simulink library "sm_excv_chassis_lib"  (R2026a)
settings: Solver=VariableStepAuto
undefined symbols (not defined in the file): Excv, Trac, track_seg_tgts_seg25i2u0r3, TracTrac, X, Y, Z
libraries: sm_lib x169, nesl_utility x12, $bdroot x8, sm_trackV_lib_chain_underc_elem x4
(part 1 of 4)
Description:
  | Copyright 2024-2026 The MathWorks, Inc.
settings Model: Creator=smiller  LastModifiedBy=smiller

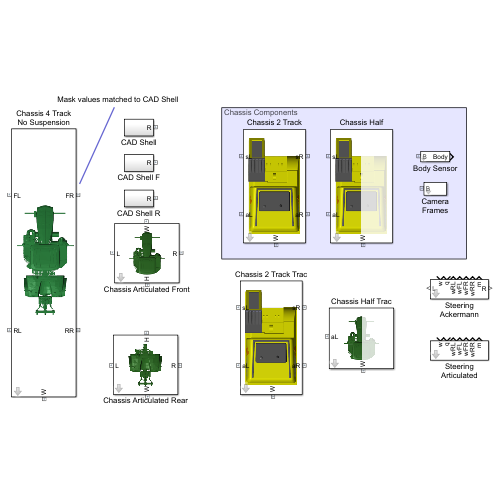
[thumbnail: Simulink's stored preview of the top-level diagram]
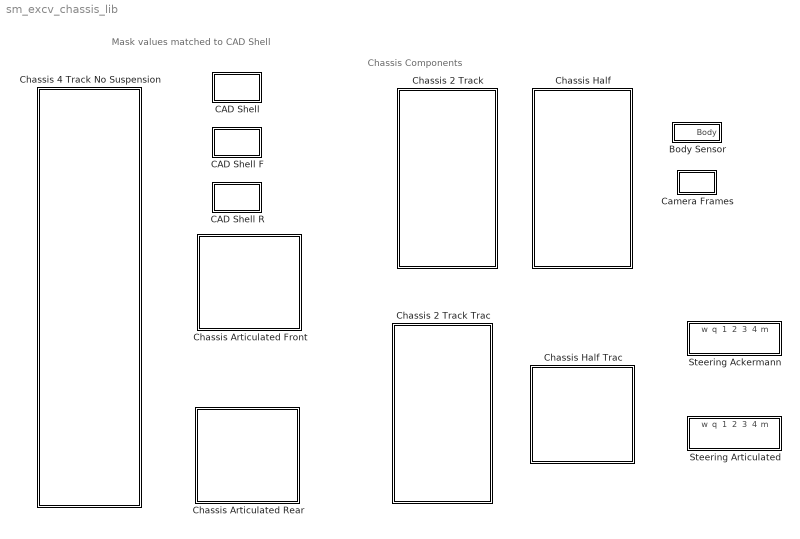
== system sm_excv_chassis_lib ==
  note: Mask values matched to CAD Shell
  note: Chassis Components
  Body Sensor : Subsystem  mask(Measurements in Body Frame){offset_body_sensor=[0 0 0]}
      mask prompts: offset_body_sensor "Sensor Frame Offset [x y z] (m)"
  CAD Shell : Subsystem
  CAD Shell F : Subsystem
  CAD Shell R : Subsystem
  Camera Frames : Subsystem  mask{Camera=Excv.Chassis.Camera}
      mask prompts: Camera "Camera Offsets (structure) (m)"
  Chassis 2 Track : Subsystem  mask{offset_cg=Excv.Chassis.CGOffset, offset_axle=Excv.Chassis.AxleOffset, offset_Lcyl=Excv.Chassis.SuspOffset, offset_sprk2axle_x=Excv.Frame.AxleX, offset_sprk2axle_y=Excv.Frame.AxleY, Camera=Excv.Chassis.Camera, track_sep_ctr=Excv.Chassis.TrackSepCtr, axle_rad=Excv.Chassis.AxleRad, axle_opc=0, chassis_mass=Excv.Chassis.Mass, chassis_moi=Excv.Chassis.MOI, chassis_poi=Excv.Chassis.POI, body_clr=[1 1 0], trim_clr=[0.4 0.4 0.4], accent_clr=[1 0.6 0], chassis_opc=1, cyl_len=Excv.Chassis.Susp.Cylinder.Cylinder.Len, cyl_rad=Excv.Chassis.Susp.Cylinder.Cylinder.Rad, cyl_mass=Excv.Chassis.Susp.Cylinder.Cylinder.Mass, piston_len=Excv.Chassis.Susp.Cylinder.Piston.Len, piston_rad=Excv.Chassis.Susp.Cylinder.Piston.Rad, piston_mass=Excv.Chassis.Susp.Cylinder.Piston.Mass, spr_k=Excv.Chassis.Susp.Cylinder.k, spr_d=Excv.Chassis.Susp.Cylinder.b, spr_xeq=Excv.Chassis.Susp.Cylinder.xeq}
      mask prompts: offset_cg "Offset to CG [long height lat] (m)"; offset_axle "Offset to Axle [long height lat] (m)"; offset_Lcyl "Offset to Left Cylinder [long height lat] (m)"; offset_sprk2axle_x "Offset Sprocket to Axle Long (m)"; offset_sprk2axle_y "Offset Sprocket to Axle Height (m)"; Camera "Camera Offsets (structure) (m)"; track_sep_ctr "Track Width (m)"; axle_rad "Axle Radius (m)"; axle_opc "Axle Opacity (0-1)"; chassis_mass "Chassis Mass (kg)"; chassis_moi "Chassis Moments of Inertia (kg*m^2)"; chassis_poi "Chassis Products of Inertia (kg*m^2)"; body_clr "Body Color [R G B] (0-1)"; trim_clr "Trim Color  [R G B] (0-1)"; accent_clr "Accent Color [R G B] (0-1)"; chassis_opc "Opacity (0-1)"; cyl_len "Cylinder Length (m)"; cyl_rad "Cylinder Radius (m)"; cyl_mass "Cylinder Mass (kg)"; piston_len "Piston Length (m)"; piston_rad "Piston Radius (m)"; piston_mass "Piston Mass (kg)"; spr_k "Stiffness (N/m)"; spr_d "Damping (N/(m/s))"; spr_xeq "Equilibrium Position (m)"
      settings: PortSchema="{\"entries\":[{\"content\":{\"sides\":[{\"content\":{\"connectorIds\":[\"LConn1\",\"LConn2\"]},\"type\":\"ConnectorPlacement.EquallySpacedRectSide\",\"uuid\":\"edd0f9cd-c75d-460e-8747-c453c06c3b51\"},{\"content\":{\"connectorIds\":[\"RConn1\",\"RConn2\"],\"side\":\"RIGHT\"},\"type\":\"ConnectorPlacement.EquallySpacedRectSide\",\"uuid\":\"aac0b74e-f978-42e3-a6a1-4bc72aaab1ab\"},{\"content\":{\"side\":\"TOP\"},\"type\":\"ConnectorPlacement.EquallySpacedRectSide\",\"uuid\":\"f25955ca-c2f5-46fd-b059-2b680dae975d\"},{\"content\":{\"connectorIds\":[\"RConn3\"],\"side\":\"BOTTOM\"},\"type\":\"ConnectorPlacement.EquallySpacedRectSide\",\"uuid\":\"7501e828-daf5-40c9-b971-42e639c94cdf\"}]},\"type\":\"ConnectorPlacement.EquallySpacedConnector\",\"uuid\":\"6826b738-8ce7-493d-aa91-65501067c2e5\"}],\"packageUris\":[\"http://schema.mathworks.com/mf0/Connector/R2020b\"],\"version\":\"1.0\"}"
      mask TypeOptions offset_cg:
      | Transform
      | Chassis Ref to CG/TranslationCartesianOffset
      mask TypeOptions offset_axle:
      | Transform
      | Chassis Ref
      | to Axle/TranslationCartesianOffset
      mask TypeOptions Camera:
      | Camera
      | Frames/Camera
      mask TypeOptions axle_rad: Axle/CylinderRadius
      mask TypeOptions axle_opc: Axle/GraphicOpacity
      mask TypeOptions chassis_mass:
      | Inertia
      | Chassis/Mass
      mask TypeOptions chassis_moi:
      | Inertia
      | Chassis/MomentsOfInertia
      mask TypeOptions chassis_poi:
      | Inertia
      | Chassis/ProductsOfInertia
      mask TypeOptions cyl_len:
      | Cylinder
      | Left/cyl_len | Cylinder
      | Right/cyl_len
      mask TypeOptions cyl_rad:
      | Cylinder
      | Left/cyl_rad | Cylinder
      | Right/cyl_rad
      mask TypeOptions cyl_mass:
      | Cylinder
      | Left/cyl_mass | Cylinder
      | Right/cyl_mass
      mask TypeOptions piston_len:
      | Cylinder
      | Left/piston_len | Cylinder
      | Right/piston_len
      mask TypeOptions piston_rad:
      | Cylinder
      | Left/piston_rad | Cylinder
      | Right/piston_rad
      mask TypeOptions piston_mass:
      | Cylinder
      | Left/piston_mass | Cylinder
      | Right/piston_mass
      mask TypeOptions spr_k:
      | Cylinder
      | Left/spr_k | Cylinder
      | Right/spr_k
      mask TypeOptions spr_d:
      | Cylinder
      | Left/spr_d | Cylinder
      | Right/spr_d
      mask TypeOptions spr_xeq:
      | Cylinder
      | Left/spr_xeq | Cylinder
      | Right/spr_xeq
      mask DialogControl tab_chassis Prompt: Chassis
      mask DialogControl cont_offset_chaRef Prompt: Offsets from Chassis Reference
      mask DialogControl cont_offset_track Prompt: Track Offsets
      mask DialogControl cont_dims Prompt: Dimensions
      mask DialogControl cont_mass Prompt: Mass and Inertia
      mask DialogControl cont_appear Prompt: Appearance
      mask DialogControl tab_susp Prompt: Suspension
      mask DialogControl cont_susp Prompt: Suspension
      mask Display: image('sm_excv_track_chassis_topview_IMAGE.png')
  Chassis 2 Track Trac : Subsystem  mask{offset_cg=Trac.Chassis.CGOffset, offset_axle=Trac.Chassis.AxleOffset, offset_Lcyl=Trac.Chassis.SuspOffset, offset_sprk2axle_x=Trac.Frame.SprkOffLon.Axle, offset_sprk2axle_y=Trac.Frame.SprkOffVer.Axle, Camera=Trac.Chassis.Camera, track_sep_ctr=Trac.Chassis.TrackSepCtr, axle_rad=Trac.Chassis.AxleRad, axle_opc=0, chassis_mass=Trac.Chassis.Mass/4, chassis_moi=Trac.Chassis.MOI/4, chassis_poi=Trac.Chassis.POI/4, cyl_len=Trac.Chassis.Susp.Cylinder.Cylinder.Len, cyl_rad=Trac.Chassis.Susp.Cylinder.Cylinder.Rad, cyl_mass=Trac.Chassis.Susp.Cylinder.Cylinder.Mass, piston_len=Trac.Chassis.Susp.Cylinder.Piston.Len, piston_rad=TracTrac.Chassis.Susp.Cylinder.Piston.Rad, piston_mass=Trac.Chassis.Susp.Cylinder.Piston.Mass, spr_k=Trac.Chassis.Susp.Cylinder.k, spr_d=track_seg_tgts_seg25i2u0r3.Chassis.Susp.Cylinder.b, spr_xeq=TracTrac.Chassis.Susp.Cylinder.xeq}
      mask prompts: offset_cg "Offset to CG [long height lat] (m)"; offset_axle "Offset to Axle [long height lat] (m)"; offset_Lcyl "Offset to Left Cylinder [long height lat] (m)"; offset_sprk2axle_x "Offset Sprocket to Axle Long (m)"; offset_sprk2axle_y "Offset Sprocket to Axle Height (m)"; Camera "Camera Offsets (structure) (m)"; track_sep_ctr "Track Width (m)"; axle_rad "Axle Radius (m)"; axle_opc "Axle Opacity (0-1)"; chassis_mass "Chassis Mass (kg)"; chassis_moi "Chassis Moments of Inertia (kg*m^2)"; chassis_poi "Chassis Products of Inertia (kg*m^2)"; cyl_len "Cylinder Length (m)"; cyl_rad "Cylinder Radius (m)"; cyl_mass "Cylinder Mass (kg)"; piston_len "Piston Length (m)"; piston_rad "Piston Radius (m)"; piston_mass "Piston Mass (kg)"; spr_k "Stiffness (N/m)"; spr_d "Damping (N/(m/s))"; spr_xeq "Equilibrium Position (m)"
      settings: PortSchema="{\"entries\":[{\"content\":{\"sides\":[{\"content\":{\"connectorIds\":[\"LConn1\",\"LConn2\"]},\"type\":\"ConnectorPlacement.EquallySpacedRectSide\",\"uuid\":\"edd0f9cd-c75d-460e-8747-c453c06c3b51\"},{\"content\":{\"connectorIds\":[\"RConn1\",\"RConn2\"],\"side\":\"RIGHT\"},\"type\":\"ConnectorPlacement.EquallySpacedRectSide\",\"uuid\":\"aac0b74e-f978-42e3-a6a1-4bc72aaab1ab\"},{\"content\":{\"side\":\"TOP\"},\"type\":\"ConnectorPlacement.EquallySpacedRectSide\",\"uuid\":\"f25955ca-c2f5-46fd-b059-2b680dae975d\"},{\"content\":{\"connectorIds\":[\"RConn3\"],\"side\":\"BOTTOM\"},\"type\":\"ConnectorPlacement.EquallySpacedRectSide\",\"uuid\":\"7501e828-daf5-40c9-b971-42e639c94cdf\"}]},\"type\":\"ConnectorPlacement.EquallySpacedConnector\",\"uuid\":\"6826b738-8ce7-493d-aa91-65501067c2e5\"}],\"packageUris\":[\"http://schema.mathworks.com/mf0/Connector/R2020b\"],\"version\":\"1.0\"}"
      mask TypeOptions offset_cg:
      | Transform
      | Chassis Ref to CG/TranslationCartesianOffset
      mask TypeOptions offset_axle:
      | Transform
      | Chassis Ref
      | to Axle/TranslationCartesianOffset
      mask TypeOptions Camera:
      | Camera
      | Frames/Camera
      mask TypeOptions axle_rad: Axle/CylinderRadius
      mask TypeOptions axle_opc: Axle/GraphicOpacity
      mask TypeOptions chassis_mass:
      | Inertia
      | Chassis/Mass
      mask TypeOptions chassis_moi:
      | Inertia
      | Chassis/MomentsOfInertia
      mask TypeOptions chassis_poi:
      | Inertia
      | Chassis/ProductsOfInertia
      mask TypeOptions cyl_len:
      | Cylinder
      | Left/cyl_len | Cylinder
      | Right/cyl_len
      mask TypeOptions cyl_rad:
      | Cylinder
      | Left/cyl_rad | Cylinder
      | Right/cyl_rad
      mask TypeOptions cyl_mass:
      | Cylinder
      | Left/cyl_mass | Cylinder
      | Right/cyl_mass
      mask TypeOptions piston_len:
      | Cylinder
      | Left/piston_len | Cylinder
      | Right/piston_len
      mask TypeOptions piston_rad:
      | Cylinder
      | Left/piston_rad | Cylinder
      | Right/piston_rad
      mask TypeOptions piston_mass:
      | Cylinder
      | Left/piston_mass | Cylinder
      | Right/piston_mass
      mask TypeOptions spr_k:
      | Cylinder
      | Left/spr_k | Cylinder
      | Right/spr_k
      mask TypeOptions spr_d:
      | Cylinder
      | Left/spr_d | Cylinder
      | Right/spr_d
      mask TypeOptions spr_xeq:
      | Cylinder
      | Left/spr_xeq | Cylinder
      | Right/spr_xeq
      mask DialogControl tab_chassis Prompt: Chassis
      mask DialogControl cont_offset_chaRef Prompt: Offsets from Chassis Reference
      mask DialogControl cont_offset_track Prompt: Track Offsets
      mask DialogControl cont_dims Prompt: Dimensions
      mask DialogControl cont_mass Prompt: Mass and Inertia
      mask DialogControl tab_susp Prompt: Suspension
      mask DialogControl cont_susp Prompt: Suspension
      mask Display: image('sm_excv_track_chassis_topview_IMAGE.png')
  Chassis 4 Track No Suspension : Subsystem  mask{popup_chassis_geo=CAD Shell}
      mask prompts: popup_chassis_geo "Chassis Geometry"
      mask init:
      | %if(popup_chassis_geo==1)
      | %    set_param([gcb '/Extrusion'],'LabelModeActiveChoice','None')
      | %    set_param([gcb '/CAD'],'LabelModeActiveChoice','Shell')
      | %elseif(popup_chassis_geo==2)
      | %    set_param([gcb '/Extrusion'],'LabelModeActiveChoice','Profile')
      | %    set_param([gcb '/CAD'],'LabelModeActiveChoice','None')    
      | %end
      settings: PortSchema="{\"entries\":[{\"content\":{\"sides\":[{\"content\":{\"connectorIds\":[\"LConn1\",\"LConn2\"]},\"type\":\"ConnectorPlacement.EquallySpacedRectSide\",\"uuid\":\"edd0f9cd-c75d-460e-8747-c453c06c3b51\"},{\"content\":{\"connectorIds\":[\"RConn1\",\"RConn2\"],\"side\":\"RIGHT\"},\"type\":\"ConnectorPlacement.EquallySpacedRectSide\",\"uuid\":\"aac0b74e-f978-42e3-a6a1-4bc72aaab1ab\"},{\"content\":{\"side\":\"TOP\"},\"type\":\"ConnectorPlacement.EquallySpacedRectSide\",\"uuid\":\"f25955ca-c2f5-46fd-b059-2b680dae975d\"},{\"content\":{\"connectorIds\":[\"RConn3\"],\"side\":\"BOTTOM\"},\"type\":\"ConnectorPlacement.EquallySpacedRectSide\",\"uuid\":\"7501e828-daf5-40c9-b971-42e639c94cdf\"}]},\"type\":\"ConnectorPlacement.EquallySpacedConnector\",\"uuid\":\"6826b738-8ce7-493d-aa91-65501067c2e5\"}],\"packageUris\":[\"http://schema.mathworks.com/mf0/Connector/R2020b\"],\"version\":\"1.0\"}"
      mask TypeOptions popup_chassis_geo: Chassis Front/popup_chassis_geo | Chassis Rear/popup_chassis_geo
      mask DialogControl tab_geometry Prompt: Geometry
      mask Display:
      | if(strcmp(get_param(gcb,'popup_chassis_geo'),'Extrusion Profile'))
      |     image('sm_tractor_chassis_topview_IMAGE.png')
      | elseif(strcmp(get_param(gcb,'popup_chassis_geo'),'CAD Shell'))
      |     image('sm_tractor_chassis_topview_CAD_IMAGE.png')
      | elseif(strcmp(get_param(gcb,'popup_chassis_geo'),'CAD Geometry'))
      |     image('sm_tractor_chassis_topview_CAD_IMAGE.png')
      | end
  Chassis Articulated Front : Subsystem  mask{offset_cg=Trac.Chassis.Front.CGOffset, offset_axle=Trac.Chassis.Front.AxleOffset, offset_hinge=Trac.Chassis.Front.HingeOffset, offset_cad=Trac.Chassis.Front.CADOffset, offset_sprk2axle_x=Trac.Frame.SprkOffLon.Axle, offset_sprk2axle_y=Trac.Frame.SprkOffVer.Axle, trackF_sep_ctr=Trac.Chassis.Front.TrackSepCtr, axle_rad=Trac.Chassis.Front.AxleRad, axle_opc=0, chassis_mass=Trac.Chassis.Front.Mass, chassis_moi=Trac.Chassis.Front.MOI, chassis_poi=Trac.Chassis.Front.POI, popup_chassis_geo=CAD Shell, chassis_xc=Trac.Chassis.Front.Visual.profile_xc, chassis_w=Trac.Chassis.Visual.wid, chassis_clr=Trac.Chassis.Visual.clr, chassis_opc=Trac.Chassis.Visual.opc}
      mask prompts: offset_cg "Offset to CG [long height lat] (m)"; offset_axle "Offset to Axle [long height lat] (m)"; offset_hinge "Offset Ref to Hinge [long lat height] (m)"; offset_cad "Offset Ref to CAD [long lat height] (m)"; offset_sprk2axle_x "Offset Sprocket to Axle Long (m)"; offset_sprk2axle_y "Offset Sprocket to Axle Height (m)"; trackF_sep_ctr "Track Separation(m)"; axle_rad "Axle Radius (m)"; axle_opc "Axle Opacity (0-1)"; chassis_mass "Chassis Mass (kg)"; chassis_moi "Chassis Moments of Inertia (kg*m^2)"; chassis_poi "Chassis Products of Inertia (kg*m^2)"; popup_chassis_geo "Chassis Geometry"; chassis_xc "Profile [x y] (m)"; chassis_w "Width (m)"; chassis_clr "Color [R G B] (0-1)"; chassis_opc "Opacity (0-1)"
      mask init:
      | if(popup_chassis_geo==1)
      |     set_param([gcb '/Extrusion'],'LabelModeActiveChoice','None')
      |     set_param([gcb '/CAD'],'LabelModeActiveChoice','Shell')
      | elseif(popup_chassis_geo==2)
      |     set_param([gcb '/Extrusion'],'LabelModeActiveChoice','Profile')
      |     set_param([gcb '/CAD'],'LabelModeActiveChoice','None')    
      | end
      settings: PortSchema="{\"entries\":[{\"content\":{\"sides\":[{\"content\":{\"connectorIds\":[\"LConn1\"]},\"type\":\"ConnectorPlacement.EquallySpacedRectSide\",\"uuid\":\"783442ce-ff8c-4ffd-985e-ad561337c504\"},{\"content\":{\"connectorIds\":[\"RConn1\"],\"side\":\"RIGHT\"},\"type\":\"ConnectorPlacement.EquallySpacedRectSide\",\"uuid\":\"e5fa2bd9-d20b-4616-b7eb-3909246815d1\"},{\"content\":{\"connectorIds\":[\"LConn2\"],\"side\":\"TOP\"},\"type\":\"ConnectorPlacement.EquallySpacedRectSide\",\"uuid\":\"f28076e6-43a3-49af-9259-01f47a067523\"},{\"content\":{\"connectorIds\":[\"RConn2\"],\"side\":\"BOTTOM\"},\"type\":\"ConnectorPlacement.EquallySpacedRectSide\",\"uuid\":\"989dc25b-126f-403c-8e6f-29b3cb3c97a8\"}]},\"type\":\"ConnectorPlacement.EquallySpacedConnector\",\"uuid\":\"6754bff4-fda0-4d0c-baf4-bb2b798cbca1\"}],\"packageUris\":[\"http://schema.mathworks.com/mf0/Connector/R2020b\"],\"version\":\"1.0\"}"
      mask TypeOptions offset_cg:
      | Transform
      | Chassis Ref to CG/TranslationCartesianOffset
      mask TypeOptions offset_axle:
      | Transform
      | Chassis Ref
      | to Axle/TranslationCartesianOffset
      mask TypeOptions offset_hinge:
      | Transform
      | Artic Hinge/TranslationCartesianOffset
      mask TypeOptions offset_cad:
      | Transform
      | CAD Offset/TranslationCartesianOffset
      mask TypeOptions axle_rad: AxleF/CylinderRadius
      mask TypeOptions axle_opc: AxleF/GraphicOpacity
      mask TypeOptions chassis_mass:
      | Inertia
      | Chassis/Mass
      mask TypeOptions chassis_moi:
      | Inertia
      | Chassis/MomentsOfInertia
      mask TypeOptions chassis_poi:
      | Inertia
      | Chassis/ProductsOfInertia
      mask TypeOptions popup_chassis_geo: CAD Shell | Extrusion Profile
      mask DialogControl tab_chassis Prompt: Chassis
      mask DialogControl cont_offset_chaRef Prompt: Offsets from Chassis Reference
      mask DialogControl cont_offset_track Prompt: Track Offsets
      mask DialogControl cont_dims Prompt: Dimensions
      mask DialogControl cont_mass Prompt: Mass and Inertia
      mask DialogControl tab_geometry Prompt: Geometry
      mask DialogControl cont_visual Prompt: Extrusion Visual
      mask Display:
      | if(strcmp(get_param(gcb,'popup_chassis_geo'),'Extrusion Profile'))
      |     image('sm_tractor_chassisF_topview_Extr_IMAGE.png')
      | elseif(strcmp(get_param(gcb,'popup_chassis_geo'),'CAD Shell'))
      |     image('sm_tractor_chassisF_topview_CAD_IMAGE.png')
      | elseif(strcmp(get_param(gcb,'popup_chassis_geo'),'CAD Geometry'))
      |     image('sm_tractor_chassisF_topview_CAD_IMAGE.png')
      | end
  Chassis Articulated Rear : Subsystem  mask{offset_cg=Trac.Chassis.Rear.CGOffset, offset_axle=Trac.Chassis.Rear.AxleOffset, offset_hinge=Trac.Chassis.Rear.HingeOffset, offset_cad=Trac.Chassis.Rear.CADOffset, offset_sprk2axle_x=Trac.Frame.SprkOffLon.Axle, offset_sprk2axle_y=Trac.Frame.SprkOffVer.Axle, trackR_sep_ctr=Trac.Chassis.Rear.TrackSepCtr, axle_rad=Trac.Chassis.Rear.AxleRad, axle_opc=0, chassis_mass=Trac.Chassis.Rear.Mass, chassis_moi=Trac.Chassis.Rear.MOI, chassis_poi=Trac.Chassis.Rear.POI, popup_chassis_geo=CAD Shell, chassis_xc=Trac.Chassis.Rear.Visual.profile_xc, chassis_w=Trac.Chassis.Visual.wid, chassis_clr=Trac.Chassis.Visual.clr, chassis_opc=Trac.Chassis.Visual.opc}
      mask prompts: offset_cg "Offset to CG [long height lat] (m)"; offset_axle "Offset to Axle [long height lat] (m)"; offset_hinge "Offset to Hinge [long lat height] (m)"; offset_cad "Offset Ref to CAD [long lat height] (m)"; offset_sprk2axle_x "Offset Sprocket to Axle Long (m)"; offset_sprk2axle_y "Offset Sprocket to Axle Height (m)"; trackR_sep_ctr "Track Separation (m)"; axle_rad "Axle Radius (m)"; axle_opc "Axle Opacity (0-1)"; chassis_mass "Chassis Mass (kg)"; chassis_moi "Chassis Moments of Inertia (kg*m^2)"; chassis_poi "Chassis Products of Inertia (kg*m^2)"; popup_chassis_geo "Chassis Geometry"; chassis_xc "Profile [x y] (m)"; chassis_w "Width (m)"; chassis_clr "Color [R G B] (0-1)"; chassis_opc "Opacity (0-1)"
      mask init:
      | if(popup_chassis_geo==1)
      |     set_param([gcb '/Extrusion'],'LabelModeActiveChoice','None')
      |     set_param([gcb '/CAD'],'LabelModeActiveChoice','Shell')
      | elseif(popup_chassis_geo==2)
      |     set_param([gcb '/Extrusion'],'LabelModeActiveChoice','Profile')
      |     set_param([gcb '/CAD'],'LabelModeActiveChoice','None')
      | end
      settings: PortSchema="{\"entries\":[{\"content\":{\"sides\":[{\"content\":{\"connectorIds\":[\"LConn1\"]},\"type\":\"ConnectorPlacement.EquallySpacedRectSide\",\"uuid\":\"3396d2e0-5642-4e2b-9e7e-e160f0171c90\"},{\"content\":{\"connectorIds\":[\"RConn1\"],\"side\":\"RIGHT\"},\"type\":\"ConnectorPlacement.EquallySpacedRectSide\",\"uuid\":\"2f3af179-4118-4eb5-9970-94e45b31ae93\"},{\"content\":{\"connectorIds\":[\"LConn2\"],\"side\":\"TOP\"},\"type\":\"ConnectorPlacement.EquallySpacedRectSide\",\"uuid\":\"8ac22486-3c02-45cc-b667-9a74f9e438f3\"},{\"content\":{\"connectorIds\":[\"RConn2\"],\"side\":\"BOTTOM\"},\"type\":\"ConnectorPlacement.EquallySpacedRectSide\",\"uuid\":\"cc087a8c-e40e-41b5-8e74-208746138e49\"}]},\"type\":\"ConnectorPlacement.EquallySpacedConnector\",\"uuid\":\"8ae313ea-c508-4d9f-81ae-04b86ccaf0cc\"}],\"packageUris\":[\"http://schema.mathworks.com/mf0/Connector/R2020b\"],\"version\":\"1.0\"}"
      mask TypeOptions offset_cg:
      | Transform
      | Chassis Ref to CG/TranslationCartesianOffset
      mask TypeOptions offset_axle:
      | Transform
      | Chassis Ref
      | to Axle/TranslationCartesianOffset
      mask TypeOptions offset_hinge:
      | Transform
      | Artic Hinge/TranslationCartesianOffset
      mask TypeOptions offset_cad:
      | Transform
      | CAD/TranslationCartesianOffset
      mask TypeOptions axle_rad: AxleR/CylinderRadius
      mask TypeOptions axle_opc: AxleR/GraphicOpacity
      mask TypeOptions chassis_mass:
      | Inertia
      | Chassis/Mass
      mask TypeOptions chassis_moi:
      | Inertia
      | Chassis/MomentsOfInertia
      mask TypeOptions chassis_poi:
      | Inertia
      | Chassis/ProductsOfInertia
      mask TypeOptions popup_chassis_geo: CAD Shell | Extrusion Profile
      mask DialogControl tab_chassis Prompt: Chassis
      mask DialogControl cont_offset_chaRef Prompt: Offsets from Chassis Reference
      mask DialogControl cont_offset_track Prompt: Track Offsets
      mask DialogControl cont_dims Prompt: Dimensions
      mask DialogControl cont_mass Prompt: Mass and Inertia
      mask DialogControl tab_geometry Prompt: Geometry
      mask DialogControl cont_visual Prompt: Extrusion Visual
      mask Display:
      | if(strcmp(get_param(gcb,'popup_chassis_geo'),'Extrusion Profile'))
      |     image('sm_tractor_chassisR_topview_Extr_IMAGE.png')
      | elseif(strcmp(get_param(gcb,'popup_chassis_geo'),'CAD Shell'))
      |     image('sm_tractor_chassisR_topview_CAD_IMAGE.png')
      | elseif(strcmp(get_param(gcb,'popup_chassis_geo'),'CAD Geometry'))
      |     image('sm_tractor_chassisR_topview_CAD_IMAGE.png')
      | end
  Chassis Half : Subsystem  mask{Camera=Excv.Chassis.Camera, offset_cg=Excv.Chassis.CGOffset, offset_axle=Excv.Chassis.AxleOffset, offset_sprk2axle_x=Excv.Frame.AxleX, offset_sprk2axle_y=Excv.Frame.AxleY, track_sep_ctr=Excv.Chassis.TrackSepCtr, chassis_mass=Excv.Chassis.Mass/2, chassis_moi=Excv.Chassis.MOI/2, chassis_poi=Excv.Chassis.POI/2}
      mask prompts: Camera "Camera Offsets (structure) (m)"; offset_cg "Offset to CG [long height lat] (m)"; offset_axle "Offset to Axle [long height lat] (m)"; offset_sprk2axle_x "Offset Sprocket to Axle Long (m)"; offset_sprk2axle_y "Offset Sprocket to Axle Height (m)"; track_sep_ctr "Track Width (m)"; chassis_mass "Chassis Mass (kg)"; chassis_moi "Chassis Moments of Inertia (kg*m^2)"; chassis_poi "Chassis Products of Inertia (kg*m^2)"
      settings: PortSchema="{\"entries\":[{\"content\":{\"sides\":[{\"content\":{\"connectorIds\":[\"LConn1\",\"LConn2\"]},\"type\":\"ConnectorPlacement.EquallySpacedRectSide\",\"uuid\":\"edd0f9cd-c75d-460e-8747-c453c06c3b51\"},{\"content\":{\"side\":\"RIGHT\"},\"type\":\"ConnectorPlacement.EquallySpacedRectSide\",\"uuid\":\"aac0b74e-f978-42e3-a6a1-4bc72aaab1ab\"},{\"content\":{\"side\":\"TOP\"},\"type\":\"ConnectorPlacement.EquallySpacedRectSide\",\"uuid\":\"f25955ca-c2f5-46fd-b059-2b680dae975d\"},{\"content\":{\"connectorIds\":[\"RConn1\"],\"side\":\"BOTTOM\"},\"type\":\"ConnectorPlacement.EquallySpacedRectSide\",\"uuid\":\"7501e828-daf5-40c9-b971-42e639c94cdf\"}]},\"type\":\"ConnectorPlacement.EquallySpacedConnector\",\"uuid\":\"6826b738-8ce7-493d-aa91-65501067c2e5\"}],\"packageUris\":[\"http://schema.mathworks.com/mf0/Connector/R2020b\"],\"version\":\"1.0\"}"
      mask TypeOptions Camera:
      | Camera
      | Frames/Camera
      mask TypeOptions offset_cg:
      | Transform
      | Chassis Ref to CG/TranslationCartesianOffset
      mask TypeOptions offset_axle:
      | Transform
      | Chassis Ref to Axle/TranslationCartesianOffset
      mask TypeOptions chassis_mass:
      | Inertia
      | Half Chassis/Mass
      mask TypeOptions chassis_moi:
      | Inertia
      | Half Chassis/MomentsOfInertia
      mask TypeOptions chassis_poi:
      | Inertia
      | Half Chassis/ProductsOfInertia
      mask DialogControl tab_chassis Prompt: Chassis
      mask DialogControl cont_offset_chaRef Prompt: Offsets from Chassis Reference
      mask DialogControl cont_offset_track Prompt: Track Offsets
      mask DialogControl cont_dims Prompt: Dimensions
      mask DialogControl cont_mass Prompt: Mass and Inertia
      mask Display: image('sm_excv_track_chassis_half_topview_IMAGE.png');
  Chassis Half Trac : Subsystem  mask{offset_cg=Trac.Chassis.Front.CGOffset + [0 0.7 0], offset_axle=Trac.Chassis.Front.AxleOffset, offset_sprk2axle_x=Trac.Frame.SprkOffLon.Axle, offset_sprk2axle_y=Trac.Frame.SprkOffVer.Axle, track_sep_ctr=Trac.Chassis.Front.TrackSepCtr, chassis_mass=Trac.Chassis.Front.Mass/2, chassis_moi=Trac.Chassis.Front.MOI/2, chassis_poi=Trac.Chassis.Front.POI/2}
      mask prompts: offset_cg "Offset to CG [long height lat] (m)"; offset_axle "Offset to Axle [long height lat] (m)"; offset_sprk2axle_x "Offset Sprocket to Axle Long (m)"; offset_sprk2axle_y "Offset Sprocket to Axle Height (m)"; track_sep_ctr "Track Width (m)"; chassis_mass "Chassis Mass (kg)"; chassis_moi "Chassis Moments of Inertia (kg*m^2)"; chassis_poi "Chassis Products of Inertia (kg*m^2)"
      settings: PortSchema="{\"entries\":[{\"content\":{\"sides\":[{\"content\":{\"connectorIds\":[\"LConn1\"]},\"type\":\"ConnectorPlacement.EquallySpacedRectSide\",\"uuid\":\"edd0f9cd-c75d-460e-8747-c453c06c3b51\"},{\"content\":{\"side\":\"RIGHT\"},\"type\":\"ConnectorPlacement.EquallySpacedRectSide\",\"uuid\":\"aac0b74e-f978-42e3-a6a1-4bc72aaab1ab\"},{\"content\":{\"side\":\"TOP\"},\"type\":\"ConnectorPlacement.EquallySpacedRectSide\",\"uuid\":\"f25955ca-c2f5-46fd-b059-2b680dae975d\"},{\"content\":{\"connectorIds\":[\"RConn1\"],\"side\":\"BOTTOM\"},\"type\":\"ConnectorPlacement.EquallySpacedRectSide\",\"uuid\":\"7501e828-daf5-40c9-b971-42e639c94cdf\"}]},\"type\":\"ConnectorPlacement.EquallySpacedConnector\",\"uuid\":\"6826b738-8ce7-493d-aa91-65501067c2e5\"}],\"packageUris\":[\"http://schema.mathworks.com/mf0/Connector/R2020b\"],\"version\":\"1.0\"}"
      mask TypeOptions offset_cg:
      | Transform
      | Chassis Ref to CG/TranslationCartesianOffset
      mask TypeOptions offset_axle:
      | Transform
      | Chassis Ref to Axle/TranslationCartesianOffset
      mask TypeOptions chassis_mass:
      | Inertia
      | Half Chassis/Mass
      mask TypeOptions chassis_moi:
      | Inertia
      | Half Chassis/MomentsOfInertia
      mask TypeOptions chassis_poi:
      | Inertia
      | Half Chassis/ProductsOfInertia
      mask DialogControl tab_chassis Prompt: Chassis
      mask DialogControl cont_offset_chaRef Prompt: Offsets from Chassis Reference
      mask DialogControl cont_offset_track Prompt: Track Offsets
      mask DialogControl cont_dims Prompt: Dimensions
      mask DialogControl cont_mass Prompt: Mass and Inertia
      mask Display: image('sm_tractor_chassisF_half_topview_CAD_IMAGE.png');
  Steering Ackermann : Subsystem  mask{yTrack=Trac.Chassis.TrackSepCtr, steerRatio=1, tcSteer=0.1, wheelbase=Trac.Chassis.AxleSeparation}
      mask prompts: yTrack "Track Width (m)"; steerRatio "Steering Ratio"; tcSteer "Steering Filter Constant (s)"; wheelbase "Wheelbase (m)"
      settings: PortSchema="{\"entries\":[{\"content\":{\"sides\":[{\"content\":{\"connectorIds\":[\"LConn1\"]},\"type\":\"ConnectorPlacement.EquallySpacedRectSide\",\"uuid\":\"65a6d75a-79bf-476b-9435-04bcf6c2ef18\"},{\"content\":{\"connectorIds\":[\"RConn1\"],\"side\":\"RIGHT\"},\"type\":\"ConnectorPlacement.EquallySpacedRectSide\",\"uuid\":\"4d91bb65-021e-4e19-8917-9509e9fd2683\"},{\"content\":{\"connectorIds\":[\"In1\",\"In2\",\"Out1\",\"Out2\",\"Out3\",\"Out4\",\"Out5\"],\"side\":\"TOP\"},\"type\":\"ConnectorPlacement.EquallySpacedRectSide\",\"uuid\":\"f7aac0ed-f2d6-4a01-9627-e78393360ed0\"}]},\"type\":\"ConnectorPlacement.EquallySpacedConnector\",\"uuid\":\"6c2d29d9-099e-4079-9b4f-de2c4ae6c2a7\"}],\"packageUris\":[\"http://schema.mathworks.com/mf0/Connector/R2020b\"],\"version\":\"1.0\"}"
  Steering Articulated : Subsystem  mask{yTrack=Trac.Chassis.Front.TrackSepCtr, steerRatio=1, tcSteer=0.1, wheelbase=Trac.Chassis.AxleSeparation}
      mask prompts: yTrack "Track Width (m)"; steerRatio "Steering Ratio"; tcSteer "Steering Filter Constant (s)"; wheelbase "Wheelbase (m)"
      settings: PortSchema="{\"entries\":[{\"content\":{\"sides\":[{\"content\":{},\"type\":\"ConnectorPlacement.EquallySpacedRectSide\",\"uuid\":\"65a6d75a-79bf-476b-9435-04bcf6c2ef18\"},{\"content\":{\"side\":\"RIGHT\"},\"type\":\"ConnectorPlacement.EquallySpacedRectSide\",\"uuid\":\"4d91bb65-021e-4e19-8917-9509e9fd2683\"},{\"content\":{\"connectorIds\":[\"In1\",\"In2\",\"Out1\",\"Out2\",\"Out3\",\"Out4\",\"Out5\"],\"side\":\"TOP\"},\"type\":\"ConnectorPlacement.EquallySpacedRectSide\",\"uuid\":\"f7aac0ed-f2d6-4a01-9627-e78393360ed0\"}]},\"type\":\"ConnectorPlacement.EquallySpacedConnector\",\"uuid\":\"6c2d29d9-099e-4079-9b4f-de2c4ae6c2a7\"}],\"packageUris\":[\"http://schema.mathworks.com/mf0/Connector/R2020b\"],\"version\":\"1.0\"}"

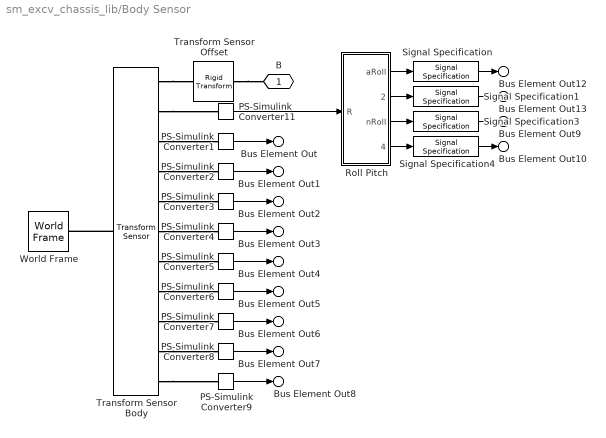
== system sm_excv_chassis_lib/Body Sensor ==
  PS-Simulink Converter1 : nesl_utility/PS-Simulink Converter  PhysicalDomain=network_engine_domain  SubClassName=ps_output  LeftPortType=input  RightPortType=output  PseudoPeriodic=off  Frequencies=[]  VectorFormat=1-D array  Unit=m  AffineConversion=off
  PS-Simulink Converter11 : nesl_utility/PS-Simulink Converter  PhysicalDomain=network_engine_domain  SubClassName=ps_output  LeftPortType=input  RightPortType=output  PseudoPeriodic=off  Frequencies=[]  VectorFormat=1-D array  Unit=1  AffineConversion=off
  PS-Simulink Converter2 : nesl_utility/PS-Simulink Converter  PhysicalDomain=network_engine_domain  SubClassName=ps_output  LeftPortType=input  RightPortType=output  PseudoPeriodic=off  Frequencies=[]  VectorFormat=1-D array  Unit=m  AffineConversion=off
  PS-Simulink Converter3 : nesl_utility/PS-Simulink Converter  PhysicalDomain=network_engine_domain  SubClassName=ps_output  LeftPortType=input  RightPortType=output  PseudoPeriodic=off  Frequencies=[]  VectorFormat=1-D array  Unit=m  AffineConversion=off
  PS-Simulink Converter4 : nesl_utility/PS-Simulink Converter  PhysicalDomain=network_engine_domain  SubClassName=ps_output  LeftPortType=input  RightPortType=output  PseudoPeriodic=off  Frequencies=[]  VectorFormat=1-D array  Unit=m/s  AffineConversion=off
  PS-Simulink Converter5 : nesl_utility/PS-Simulink Converter  PhysicalDomain=network_engine_domain  SubClassName=ps_output  LeftPortType=input  RightPortType=output  PseudoPeriodic=off  Frequencies=[]  VectorFormat=1-D array  Unit=m/s  AffineConversion=off
  PS-Simulink Converter6 : nesl_utility/PS-Simulink Converter  PhysicalDomain=network_engine_domain  SubClassName=ps_output  LeftPortType=input  RightPortType=output  PseudoPeriodic=off  Frequencies=[]  VectorFormat=1-D array  Unit=m/s  AffineConversion=off
  PS-Simulink Converter7 : nesl_utility/PS-Simulink Converter  PhysicalDomain=network_engine_domain  SubClassName=ps_output  LeftPortType=input  RightPortType=output  PseudoPeriodic=off  Frequencies=[]  VectorFormat=1-D array  Unit=m/s^2  AffineConversion=off
  PS-Simulink Converter8 : nesl_utility/PS-Simulink Converter  PhysicalDomain=network_engine_domain  SubClassName=ps_output  LeftPortType=input  RightPortType=output  PseudoPeriodic=off  Frequencies=[]  VectorFormat=1-D array  Unit=m/s^2  AffineConversion=off
  PS-Simulink Converter9 : nesl_utility/PS-Simulink Converter  PhysicalDomain=network_engine_domain  SubClassName=ps_output  LeftPortType=input  RightPortType=output  PseudoPeriodic=off  Frequencies=[]  VectorFormat=1-D array  Unit=m/s^2  AffineConversion=off
  Roll Pitch : Subsystem
  Signal Specification : SignalSpecification  Unit=rad
  Signal Specification1 : SignalSpecification  Unit=rad
  Signal Specification3 : SignalSpecification  Unit=rad/s
  Signal Specification4 : SignalSpecification  Unit=rad/s
  Transform Sensor Offset : sm_lib/Frames and Transforms/Rigid Transform  RotationMethod=None  FollAlignAxisA=+X  BaseAlignAxisA=+Y  FollAlignAxisB=+Y  BaseAlignAxisB=+Z  RotationStandardAxis=+Z  RotationAngle=0.0  RotationAngleUnits=deg  RotationArbitraryAxis=[0 0 1]  RotationSequenceAxes=FollowerAxes  RotationSequence=XYX  RotationSequenceAngles=[0 0 0]  RotationSequenceAnglesUnits=deg  RotationMatrix=[1 0 0; 0 1 0; 0 0 1]  Quaternion=[1 0 0 0]  TranslationMethod=Cartesian  TranslationCartesianOffset=offset_body_sensor  TranslationCartesianOffsetUnits=m  TranslationStandardAxis=+Z  TranslationStandardOffset=0  TranslationStandardOffsetUnits=m  TranslationROffset=0  TranslationROffsetUnits=m  TranslationThetaOffset=0  TranslationThetaOffsetUnits=deg  TranslationZOffset=0  TranslationZOffsetUnits=m
  Transform Sensor Body : sm_lib/Frames and Transforms/Transform Sensor  MeasurementFrame=NonRotatingFollower  RotationSequence=XYX  SenseAngle=off  SenseAxis=off  SenseQ=off  SenseR=on  SenseRotationSequence=off  SenseOmegaX=off  SenseOmegaY=off  SenseOmegaZ=off  SenseOmega=off  SenseQDot=off  SenseRDot=off  SenseRotationSequenceDot=off  SenseAlphaX=off  SenseAlphaY=off  SenseAlphaZ=off  SenseAlpha=off  SenseQDDot=off  SenseRDDot=off  SenseX=on  SenseY=on  SenseZ=on  SenseXYZ=off  SenseRad=off  SenseAzim=off  SenseDist=off  SenseInc=off  SenseXDot=on  SenseYDot=on  SenseZDot=on  SenseXYZDot=off  SenseRadDot=off  SenseAzimDot=off  SenseDistDot=off  SenseIncDot=off  SenseXDDot=on  SenseYDDot=on  SenseZDDot=on  SenseXYZDDot=off  SenseRadDDot=off  SenseAzimDDot=off  SenseDistDDot=off  SenseIncDDot=off
  World Frame : sm_lib/Frames and Transforms/World Frame
  B : PMIOPort  Side=Left
  Bus Element Out : Outport  VectorParamsAs1DForOutWhenUnconnected=off  PortName=Body  Element=x
  Bus Element Out1 : Outport  VectorParamsAs1DForOutWhenUnconnected=off  PortName=Body  Element=y
  Bus Element Out2 : Outport  VectorParamsAs1DForOutWhenUnconnected=off  PortName=Body  Element=z
  Bus Element Out3 : Outport  VectorParamsAs1DForOutWhenUnconnected=off  PortName=Body  Element=vx
  Bus Element Out4 : Outport  VectorParamsAs1DForOutWhenUnconnected=off  PortName=Body  Element=vy
  Bus Element Out5 : Outport  VectorParamsAs1DForOutWhenUnconnected=off  PortName=Body  Element=vz
  Bus Element Out6 : Outport  VectorParamsAs1DForOutWhenUnconnected=off  PortName=Body  Element=gx
  Bus Element Out7 : Outport  VectorParamsAs1DForOutWhenUnconnected=off  PortName=Body  Element=gy
  Bus Element Out8 : Outport  VectorParamsAs1DForOutWhenUnconnected=off  PortName=Body  Element=gz
  Bus Element Out9 : Outport  VectorParamsAs1DForOutWhenUnconnected=off  PortName=Body  Element=nRoll
  Bus Element Out10 : Outport  VectorParamsAs1DForOutWhenUnconnected=off  PortName=Body  Element=nPitch
  Bus Element Out12 : Outport  VectorParamsAs1DForOutWhenUnconnected=off  PortName=Body  Element=aRoll
  Bus Element Out13 : Outport  VectorParamsAs1DForOutWhenUnconnected=off  PortName=Body  Element=aPitch
  wires:
  PS-Simulink Converter9/1 -> Bus Element Out8/1
  PS-Simulink Converter11/1 -> Roll Pitch/1(R)
  PS-Simulink Converter6/1 -> Bus Element Out5/1
  PS-Simulink Converter7/1 -> Bus Element Out6/1
  PS-Simulink Converter2/1 -> Bus Element Out1/1
  PS-Simulink Converter8/1 -> Bus Element Out7/1
  PS-Simulink Converter5/1 -> Bus Element Out4/1
  PS-Simulink Converter3/1 -> Bus Element Out2/1
  PS-Simulink Converter1/1 -> Bus Element Out/1
  PS-Simulink Converter4/1 -> Bus Element Out3/1
  Signal Specification/1 -> Bus Element Out12/1
  Signal Specification1/1 -> Bus Element Out13/1
  Signal Specification3/1 -> Bus Element Out9/1
  Signal Specification4/1 -> Bus Element Out10/1
  Roll Pitch/3(nRoll) -> Signal Specification3/1
  Roll Pitch/4(nPitch) -> Signal Specification4/1
  Roll Pitch/2(aPitch) -> Signal Specification1/1
  Roll Pitch/1(aRoll) -> Signal Specification/1
  connections:
  Transform Sensor Body/RConn5 -- PS-Simulink Converter3/LConn1
  Transform Sensor Body/RConn4 -- PS-Simulink Converter2/LConn1
  Transform Sensor Body/RConn11 -- PS-Simulink Converter9/LConn1
  Transform Sensor Body/RConn2 -- PS-Simulink Converter11/LConn1
  Transform Sensor Body/RConn7 -- PS-Simulink Converter5/LConn1
  Transform Sensor Body/RConn3 -- PS-Simulink Converter1/LConn1
  Transform Sensor Body/LConn1 -- World Frame/RConn1
  Transform Sensor Offset/LConn1 -- B/RConn1
  Transform Sensor Body/RConn10 -- PS-Simulink Converter8/LConn1
  Transform Sensor Body/RConn9 -- PS-Simulink Converter7/LConn1
  Transform Sensor Body/RConn8 -- PS-Simulink Converter6/LConn1
  Transform Sensor Body/RConn6 -- PS-Simulink Converter4/LConn1
  Transform Sensor Body/RConn1 -- Transform Sensor Offset/RConn1

== system sm_excv_chassis_lib/CAD Shell ==
  File Solid : sm_lib/Body Elements/File Solid  ExtGeomFileName=tractor_chassis.stl  UnitType=Custom  ExtGeomFileUnits=mm  StepReaderType=HEX  ExportConvexHullGeometry=off  InertiaType=PointMass  BasedOnType=DensityFromFile  Density=1000  DensityUnits=kg/m^3  Mass=0  MassUnits=kg  CenterOfMass=[0 0 0]  CenterOfMassUnits=m  MomentsOfInertia=[1 1 1]  MomentsOfInertiaUnits=kg*m^2  ProductsOfInertia=[0 0 0]  ProductsOfInertiaUnits=kg*m^2  GraphicType=FromGeometry  MarkerShape=Sphere  MarkerSize=10  GraphicVisPropType=SimpleVisualProperties  GraphicDiffuseColor=Trac.Chassis.Visual.clr  GraphicOpacity=1.0  GraphicSpecularColor=[0.5 0.5 0.5 1.0]  GraphicAmbientColor=[0.15 0.15 0.15 1.0]  GraphicEmissiveColor=[0.0 0.0 0.0 1.0]  GraphicShininess=75  DoExposeReferenceFrame=on  SerializedFrames=<Frames/>
  Rigid Transform : sm_lib/Frames and Transforms/Rigid Transform  RotationMethod=RotationSequence  FollAlignAxisA=+X  BaseAlignAxisA=+Y  FollAlignAxisB=+Y  BaseAlignAxisB=+Z  RotationStandardAxis=+Z  RotationAngle=90  RotationAngleUnits=deg  RotationArbitraryAxis=[0 0 1]  RotationSequenceAxes=FollowerAxes  RotationSequence=ZYX  RotationSequenceAngles=[90 0 90]  RotationSequenceAnglesUnits=deg  RotationMatrix=[1 0 0; 0 1 0; 0 0 1]  Quaternion=[1 0 0 0]  TranslationMethod=Cartesian  TranslationCartesianOffset=[2.325 0 -1.35]  TranslationCartesianOffsetUnits=m  TranslationStandardAxis=+Z  TranslationStandardOffset=0  TranslationStandardOffsetUnits=m  TranslationROffset=0  TranslationROffsetUnits=m  TranslationThetaOffset=0  TranslationThetaOffsetUnits=deg  TranslationZOffset=0  TranslationZOffsetUnits=m
  R : PMIOPort  Side=Right
  connections:
  File Solid/RConn1 -- Rigid Transform/RConn1
  Rigid Transform/LConn1 -- R/RConn1

== system sm_excv_chassis_lib/CAD Shell F ==
  File Solid : sm_lib/Body Elements/File Solid  ExtGeomFileName=tractor_chassis_front.stl  UnitType=Custom  ExtGeomFileUnits=mm  StepReaderType=HEX  ExportConvexHullGeometry=off  InertiaType=PointMass  BasedOnType=DensityFromFile  Density=1000  DensityUnits=kg/m^3  Mass=0  MassUnits=kg  CenterOfMass=[0 0 0]  CenterOfMassUnits=m  MomentsOfInertia=[1 1 1]  MomentsOfInertiaUnits=kg*m^2  ProductsOfInertia=[0 0 0]  ProductsOfInertiaUnits=kg*m^2  GraphicType=FromGeometry  MarkerShape=Sphere  MarkerSize=10  GraphicVisPropType=SimpleVisualProperties  GraphicDiffuseColor=Trac.Chassis.Visual.clr  GraphicOpacity=1.0  GraphicSpecularColor=[0.5 0.5 0.5 1.0]  GraphicAmbientColor=[0.15 0.15 0.15 1.0]  GraphicEmissiveColor=[0.0 0.0 0.0 1.0]  GraphicShininess=75  DoExposeReferenceFrame=on  SerializedFrames=<Frames/>
  Rigid Transform : sm_lib/Frames and Transforms/Rigid Transform  RotationMethod=RotationSequence  FollAlignAxisA=+X  BaseAlignAxisA=+Y  FollAlignAxisB=+Y  BaseAlignAxisB=+Z  RotationStandardAxis=+Z  RotationAngle=90  RotationAngleUnits=deg  RotationArbitraryAxis=[0 0 1]  RotationSequenceAxes=FollowerAxes  RotationSequence=ZYX  RotationSequenceAngles=[90 0 90]  RotationSequenceAnglesUnits=deg  RotationMatrix=[1 0 0; 0 1 0; 0 0 1]  Quaternion=[1 0 0 0]  TranslationMethod=Cartesian  TranslationCartesianOffset=[2.325 0 -1.35]  TranslationCartesianOffsetUnits=m  TranslationStandardAxis=+Z  TranslationStandardOffset=0  TranslationStandardOffsetUnits=m  TranslationROffset=0  TranslationROffsetUnits=m  TranslationThetaOffset=0  TranslationThetaOffsetUnits=deg  TranslationZOffset=0  TranslationZOffsetUnits=m
  R : PMIOPort  Side=Right
  connections:
  Rigid Transform/LConn1 -- R/RConn1
  File Solid/RConn1 -- Rigid Transform/RConn1

== system sm_excv_chassis_lib/CAD Shell R ==
  File Solid : sm_lib/Body Elements/File Solid  ExtGeomFileName=tractor_chassis_rear.stl  UnitType=Custom  ExtGeomFileUnits=mm  StepReaderType=HEX  ExportConvexHullGeometry=off  InertiaType=PointMass  BasedOnType=DensityFromFile  Density=1000  DensityUnits=kg/m^3  Mass=0  MassUnits=kg  CenterOfMass=[0 0 0]  CenterOfMassUnits=m  MomentsOfInertia=[1 1 1]  MomentsOfInertiaUnits=kg*m^2  ProductsOfInertia=[0 0 0]  ProductsOfInertiaUnits=kg*m^2  GraphicType=FromGeometry  MarkerShape=Sphere  MarkerSize=10  GraphicVisPropType=SimpleVisualProperties  GraphicDiffuseColor=Trac.Chassis.Visual.clr  GraphicOpacity=1.0  GraphicSpecularColor=[0.5 0.5 0.5 1.0]  GraphicAmbientColor=[0.15 0.15 0.15 1.0]  GraphicEmissiveColor=[0.0 0.0 0.0 1.0]  GraphicShininess=75  DoExposeReferenceFrame=on  SerializedFrames=<Frames/>
  Rigid Transform : sm_lib/Frames and Transforms/Rigid Transform  RotationMethod=RotationSequence  FollAlignAxisA=+X  BaseAlignAxisA=+Y  FollAlignAxisB=+Y  BaseAlignAxisB=+Z  RotationStandardAxis=+Z  RotationAngle=90  RotationAngleUnits=deg  RotationArbitraryAxis=[0 0 1]  RotationSequenceAxes=FollowerAxes  RotationSequence=ZYX  RotationSequenceAngles=[90 0 90]  RotationSequenceAnglesUnits=deg  RotationMatrix=[1 0 0; 0 1 0; 0 0 1]  Quaternion=[1 0 0 0]  TranslationMethod=Cartesian  TranslationCartesianOffset=[2.325 0 -1.35]  TranslationCartesianOffsetUnits=m  TranslationStandardAxis=+Z  TranslationStandardOffset=0  TranslationStandardOffsetUnits=m  TranslationROffset=0  TranslationROffsetUnits=m  TranslationThetaOffset=0  TranslationThetaOffsetUnits=deg  TranslationZOffset=0  TranslationZOffsetUnits=m
  R : PMIOPort  Side=Right
  connections:
  File Solid/RConn1 -- Rigid Transform/RConn1
  Rigid Transform/LConn1 -- R/RConn1
